simulink model "Assignment_3_simulink"  (R2025a)
settings: Solver=FixedStepDiscrete  StartTime=0.0  StopTime=inf  FixedStep=0.1  RelTol=1e-3  EnableMultiTasking=on
model workspace (MAT data in the model file):
  SL_ROS_VariableLengthArrays_MaxSizes.CommonInfo.ArrayTruncateAction = 'EmitWarning'
  SL_ROS_VariableLengthArrays_MaxSizes.MsgTypeMap = containers.Map
  SL_ROS_VariableLengthArrays_MaxSizes.MsgTypeMap.serialization.keys = {'sensor_msgs/Image', 'sensor_msgs/LaserScan'}
  SL_ROS_VariableLengthArrays_MaxSizes.MsgTypeMap.serialization.values{1}(1).PropertyName = 'data'
  SL_ROS_VariableLengthArrays_MaxSizes.MsgTypeMap.serialization.values{1}(1).DataType = 'uint8'
  SL_ROS_VariableLengthArrays_MaxSizes.MsgTypeMap.serialization.values{1}(1).MaxLength = 921600
  SL_ROS_VariableLengthArrays_MaxSizes.MsgTypeMap.serialization.values{1}(2).PropertyName = 'encoding'
  SL_ROS_VariableLengthArrays_MaxSizes.MsgTypeMap.serialization.values{1}(2).DataType = 'uint8'
  SL_ROS_VariableLengthArrays_MaxSizes.MsgTypeMap.serialization.values{1}(2).MaxLength = 128
  SL_ROS_VariableLengthArrays_MaxSizes.MsgTypeMap.serialization.values{2}(1).PropertyName = 'intensities'
  SL_ROS_VariableLengthArrays_MaxSizes.MsgTypeMap.serialization.values{2}(1).DataType = 'single'
  SL_ROS_VariableLengthArrays_MaxSizes.MsgTypeMap.serialization.values{2}(1).MaxLength = 360
  SL_ROS_VariableLengthArrays_MaxSizes.MsgTypeMap.serialization.values{2}(2).PropertyName = 'ranges'
  SL_ROS_VariableLengthArrays_MaxSizes.MsgTypeMap.serialization.values{2}(2).DataType = 'single'
  SL_ROS_VariableLengthArrays_MaxSizes.MsgTypeMap.serialization.values{2}(2).MaxLength = 360
  SL_ROS_VariableLengthArrays_MaxSizes.MsgTypeMap.serialization.uniformity = 0
  SL_ROS_VariableLengthArrays_MaxSizes.MsgTypeMap.serialization.keyType = 'char'
  SL_ROS_VariableLengthArrays_MaxSizes.MsgTypeMap.serialization.valueType = 'any'
values from neighbouring files (symbols this model uses):
  Kv = 0.8    [Assignment_3.m]
  Kw = 0.3    [Assignment_3.m]
  limit_inf = zeros(1,length(hsv_1))    [Assignment_3.m]
  limit_sup = zeros(1,length(hsv_1))    [Assignment_3.m]
  theta_ref = 1.05*pi    (= 3.29867228627)    [Assignment_3.m]
  toll = 0.001    [Assignment_3.m]
undefined symbols (not defined in the file or in its folder): Rec, SDTV, twist
libraries: ros2lib x6, simulink x3, visionstatistics x1, visionconversions x1, visiontextngfix x1
settings Model: Creator=diego  LastModifiedBy=nicola-bertocchi
settings OptimizationCC: DefaultParameterBehavior=Inlined  EnhancedBackFolding=on  PassReuseOutputArgsAs=Individual arguments  ZeroExternalMemoryAtStartup=off  ZeroInternalMemoryAtStartup=off  MaxStackSize=64  OptimizeBlockOrder=speed  DifferentSizesBufferReuse=on  OptimizationCustomize=off  EfficientTunableParamExpr=on
settings DebuggingCC: ParameterTunabilityLossMsg=error
settings HardwareCC: ProdBitPerLong=64.0  ProdHWDeviceType=Intel->x86-64 (Linux 64)
settings SFSimCC: MATLABDynamicMemAlloc=off
settings RTWCC: SystemTargetFile=ert.tlc  HardwareBoard=Robot Operating System 2 (ROS 2)  TLCOptions="-aInlineSetEventsForThisBaseRateFcn=TLC_FALSE -aSuppressMultiTaskScheduler=TLC_FALSE  -aRateBasedStepFcn=0"  TemplateMakefile=ert_default_tmf  Toolchain=Colcon Tools  TargetLang=C++  Description=Embedded Coder
settings CodeAppCC: ForceParamTrailComments=on  IgnoreCustomStorageClasses=off  OperatorAnnotations=on  SimulinkDataObjDesc=on  SFDataObjDesc=on  InsertBlockDesc=on
settings ERTTargetCC: ExtModeTransport=2.0  ExtModeAutomaticAllocSize=off  RootIOFormat=Structure reference  CodeInterfacePackaging=C++ class

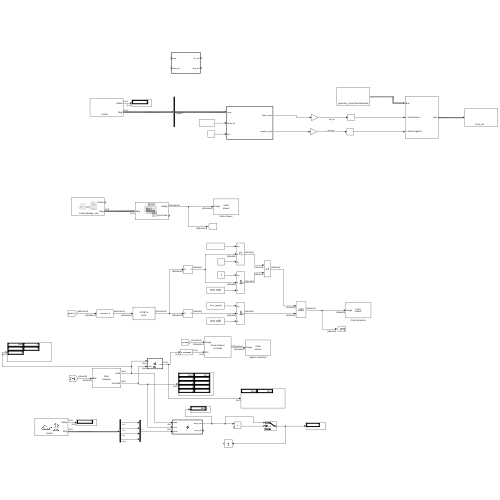
[thumbnail: Simulink's stored preview of the top-level diagram]
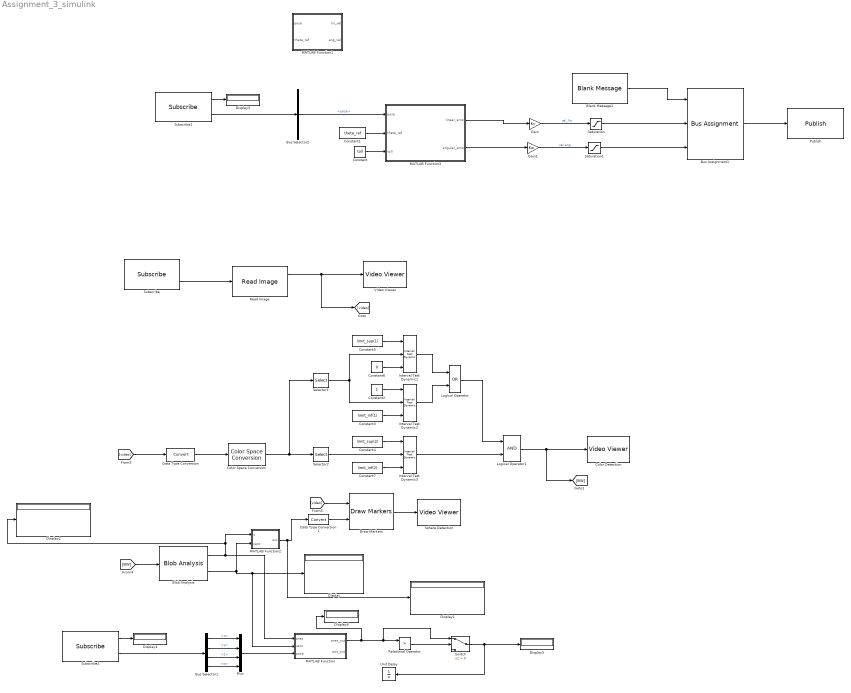
== system Assignment_3_simulink ==
  Blank Message1 : ros2lib/Blank Message  messageClass=Message  entityType=geometry_msgs/TwistStamped  messageType=geometry_msgs/TwistStamped  SampleTime=inf
  Blob Analysis : visionstatistics/Blob Analysis  Tag=vipblks_row_conv  area=on  centroid=on  bBox=off  majorAxis=off  minorAxis=off  angle=off  eccentricity=off  equivDiameterSq=off  extent=off  perimeter=off  outDT=double  conn=8  isLabel=off  maxBlobs=5  warnIfNumBlobsExceeded=on  isCount=off  useMinArea=off  minArea=0  useMaxArea=off  maxArea=intmax('uint32')  excludeBorderBlob=off  isOutVarDim=off  isFill=on  fillValues=-1  roundingMode=Floor  overflowMode=off  prodOutputMode=Binary point scaling  prodOutputWordLength=32  prodOutputFracLength=16  accumMode=Binary point scaling  accumWordLength=32  accumFracLength=0  outputMode=Binary point scaling  outputWordLength=32  outputFracLength=16  firstCoeffMode=Binary point scaling  firstCoeffWordLength=16  firstCoeffFracLength=14  secondCoeffMode=Binary point scaling  secondCoeffWordLength=32  secondCoeffFracLength=16
  Bus Assignment1 : BusAssignment  AssignedSignals=twist.linear.x,twist.angular.z
  Bus Selector1 : BusSelector  OutputSignals=pose.pose.orientation.x,pose.pose.orientation.y,pose.pose.orientation.z,pose.pose.orientation.w
  Bus Selector2 : BusSelector  OutputSignals=pose
  Color Detection : VideoViewer  FigPos=[915 518 418 304]
  Color Space Conversion : visionconversions/Color Space  Conversion  conversion=Obsolete  conversionActive=R'G'B' to HSV  wp_str=D65  rec=Rec. 601 (SDTV)  sys=1125/60/2:1  imagePorts=One multidimensional signal
  Constant : Constant  Value=toll
  Constant1 : Constant  Value=theta_ref
  Constant2 : Constant
  Constant3 : Constant  Value=limit_inf(1)
  Constant4 : Constant  Value=limit_sup(2)
  Constant5 : Constant  Value=limit_sup(1)
  Constant6 : Constant  Value=0
  Constant7 : Constant  Value=limit_inf(2)
  Data Type Conversion : DataTypeConversion  SaturateOnIntegerOverflow=off  RndMeth=Floor
  Data Type Conversion1 : DataTypeConversion  SaturateOnIntegerOverflow=off  RndMeth=Floor
  Display{,1..6} (7 alike) : Display
  Draw Markers : visiontextngfix/Draw Markers  shape=X-mark  size=25  fill=off  fillClrSource=Specify via dialog  display=User-specified value  intensity=200  color=[255 0 0]  opacity=0.6  viewport=Entire image  antialiasing=off  inType=Obsolete  imagePorts=One multidimensional signal  roundingMode=Floor  overflowMode=off  memoryMode=Specify word length  memoryWordLength=16  memoryFracLength=15  prodOutputMode=Binary point scaling  prodOutputWordLength=32  prodOutputFracLength=14
  Gain : Gain  Gain=Kv
  Gain1 : Gain  Gain=Kw
  Interval Test Dynamic1 : simulink/Logic and Bit Operations/Interval Test Dynamic  IntervalClosedRight=on  IntervalClosedLeft=on  OutDataTypeStr=boolean
  Interval Test Dynamic2 : simulink/Logic and Bit Operations/Interval Test Dynamic  IntervalClosedRight=on  IntervalClosedLeft=on  OutDataTypeStr=boolean
  Interval Test Dynamic3 : simulink/Logic and Bit Operations/Interval Test Dynamic  IntervalClosedRight=on  IntervalClosedLeft=on  OutDataTypeStr=boolean
  Logical Operator : Logic  Operator=OR  AllPortsSameDT=off  OutDataTypeStr=boolean
  Logical Operator1 : Logic  AllPortsSameDT=off  OutDataTypeStr=boolean
  MATLAB Function : MATLAB Function  TreatAsAtomicUnit=on
  MATLAB Function1 : MATLAB Function  TreatAsAtomicUnit=on
  MATLAB Function2 : MATLAB Function  TreatAsAtomicUnit=on
  MATLAB Function3 : MATLAB Function  TreatAsAtomicUnit=on
  Mux : Mux
  Publish : ros2lib/Publish  topicSource=Select from ROS network  topic=/cmd_vel  messageType=geometry_msgs/TwistStamped  QOSHistory=Keep last  QOSDepth=10  QOSReliability=Reliable  QOSDurability=Volatile  QOSDeadline=Inf  QOSLifespan=Inf  QOSLiveliness=Automatic  QOSLeaseDuration=Inf  QOSAvoidROSNamespaceConventions=off
  Read Image : ros2lib/Read Image  MaximumImageSize=[480, 640]  ImageEncoding=rgb8  ShowAlphaOutput=off  ShowErrorCodeOutput=on  VariableSizeOutputs=off
  Relational Operator : RelationalOperator  Operator=>  OutDataTypeStr=boolean  RndMeth=Simplest  InputSameDT=off
  Saturation : Saturate  UpperLimit=0.2  LowerLimit=0
  Saturation1 : Saturate  UpperLimit=0.4  LowerLimit=0
  Selector1 : Selector  NumberOfDimensions=3  InputPortWidth=3  IndexOptions=Index vector (dialog),Index vector (dialog),Index vector (dialog)  Indices=[1:480],[1:640],1  OutputSizes=1,1,1
  Selector2 : Selector  NumberOfDimensions=3  InputPortWidth=3  IndexOptions=Index vector (dialog),Index vector (dialog),Index vector (dialog)  Indices=[1:480],[1:640],2  OutputSizes=1,1,1
  Sphere Detection : VideoViewer  FigPos=[795 742 511 303]
  Subscribe : ros2lib/Subscribe  topicSource=Select from ROS network  topic=/camera/image_raw  messageType=sensor_msgs/Image  sampleTime=-1  QOSHistory=Keep last  QOSDepth=10  QOSReliability=Reliable  QOSDurability=Volatile  QOSDeadline=Inf  QOSLifespan=Inf  QOSLiveliness=Automatic  QOSLeaseDuration=Inf  QOSAvoidROSNamespaceConventions=off
  Subscribe1 : ros2lib/Subscribe  topicSource=Select from ROS network  topic=/odom  messageType=nav_msgs/Odometry  sampleTime=-1  QOSHistory=Keep last  QOSDepth=10  QOSReliability=Reliable  QOSDurability=Volatile  QOSDeadline=Inf  QOSLifespan=Inf  QOSLiveliness=Automatic  QOSLeaseDuration=Inf  QOSAvoidROSNamespaceConventions=off
  Subscribe2 : ros2lib/Subscribe  topicSource=Select from ROS network  topic=/odom  messageType=nav_msgs/Odometry  sampleTime=-1  QOSHistory=Keep last  QOSDepth=10  QOSReliability=Reliable  QOSDurability=Volatile  QOSDeadline=Inf  QOSLifespan=Inf  QOSLiveliness=Automatic  QOSLeaseDuration=Inf  QOSAvoidROSNamespaceConventions=off
  Switch : Switch  Criteria=u2 > Threshold  SaturateOnIntegerOverflow=off  InputSameDT=off
  Unit Delay : UnitDelay  SampleTime=-1  HasFrameUpgradeWarning=on
  Video Viewer : VideoViewer  FigPos=[155 894 418 304]
  wires:
  Subscribe/2 -> Read Image/1
  Read Image/1 -> Video Viewer/1, [video]
  [video] -> Data Type Conversion/1
  Data Type Conversion/1 -> Color Space Conversion/1
  Color Space Conversion/1 -> Selector1/1, Selector2/1
  [BW] -> Blob Analysis/1
  Blob Analysis/1 -> MATLAB Function2/1(u), Display2/1, MATLAB Function/1(area)
  MATLAB Function2/1(out) -> Display1/1, Data Type Conversion1/1
  Blob Analysis/2 -> MATLAB Function/2(cent), Display/1, MATLAB Function2/2(cent)
  Data Type Conversion1/1 -> Draw Markers/2
  [video] -> Draw Markers/1
  Draw Markers/1 -> Sphere Detection/1
  Bus Assignment1/1 -> Publish/1
  Gain/1 -> Saturation/1  "vel_lin"
  Gain1/1 -> Saturation1/1  "vel ang"
  Saturation1/1 -> Bus Assignment1/3
  Subscribe1/1 -> Display3/1
  Saturation/1 -> Bus Assignment1/2
  Subscribe1/2 -> Bus Selector2/1
  Bus Selector2/1 -> MATLAB Function3/1(pose)  "<pose>"
  Blank Message1/1 -> Bus Assignment1/1
  Constant1/1 -> MATLAB Function3/2(theta_ref)
  MATLAB Function3/1(linear_error) -> Gain/1
  MATLAB Function3/2(angular_error) -> Gain1/1
  Constant6/1 -> Interval Test Dynamic1/3
  Constant5/1 -> Interval Test Dynamic1/1
  Constant2/1 -> Interval Test Dynamic2/1
  Constant3/1 -> Interval Test Dynamic2/3
  Interval Test Dynamic1/1 -> Logical Operator/1
  Interval Test Dynamic2/1 -> Logical Operator/2
  Selector1/1 -> Interval Test Dynamic1/2, Interval Test Dynamic2/2
  Constant7/1 -> Interval Test Dynamic3/3
  Constant4/1 -> Interval Test Dynamic3/1
  Selector2/1 -> Interval Test Dynamic3/2
  Logical Operator/1 -> Logical Operator1/1
  Logical Operator1/1 -> [BW], Color Detection/1
  Interval Test Dynamic3/1 -> Logical Operator1/2
  Constant/1 -> MATLAB Function3/3(toll)
  Subscribe2/1 -> Display4/1
  Subscribe2/2 -> Bus Selector1/1
  MATLAB Function/1(area_out) -> Display6/1, Switch/1, Relational Operator/1
  Relational Operator/1 -> Switch/2
  Switch/1 -> Display5/1, Unit Delay/1
  Bus Selector1/1 -> Mux/1  "<x>"
  Bus Selector1/2 -> Mux/2  "<y>"
  Bus Selector1/3 -> Mux/3  "<z>"
  Bus Selector1/4 -> Mux/4  "<w>"
  Mux/1 -> MATLAB Function/3(pose)

== matlab function Assignment_3_simulink/MATLAB Function2 ==
  data: u input; out output; cent input
function out = fcn(u,cent)

[~,i] = max(u);

if ~isempty(i)
    out=cent(i,:);
else
    out=[0,0];

end

== matlab function Assignment_3_simulink/MATLAB Function ==
  data: area input; cent input; area_out output; pose input; pos_out output
function [area_out,pos_out] = fcn(area,cent,pose)

area_out = 0;
pos_out = zeros(size(pose));
[val,i] = max(area);    

if val~=-1
    if ~isempty(i)
        if cent(i,1)>315 && cent(i,1)<325
            area_out = double(val);
            pos_out = pose;
        end
    end 
end

== matlab function Assignment_3_simulink/MATLAB Function3 ==
  data: linear_error output; pose input; theta_ref input; toll input; angular_error output
function [linear_error, angular_error] = Interruttore(pose, theta_ref, toll)
    
  
 %   angular_error = 0; % Valore di default (risolve l'errore Coder)
linear_error = 0;
    q_current = [pose.pose.orientation.x; 
                 pose.pose.orientation.y; 
                 pose.pose.orientation.z; 
                 pose.pose.orientation.w];
             
% 1. Definisci l'input (Yaw, Pitch, Roll)
eul = [theta_ref, 0, 0]; 

% 2. Chiama la funzione. L'output è [w, x, y, z]
q_matlab = eul2quat(eul); 

% 3. Riordina l'output nel formato ROS [x, y, z, w]
q_target = [q_matlab(2);   % x
            q_matlab(3);   % y
            q_matlab(4);   % z
            q_matlab(1)];  % w

           
       % ... (Calcolo del quaternione di errore, come prima) ...
       q_current_inv = [-q_current(1); -q_current(2); -q_current(3); q_current(4)];
       x1 = q_target(1); y1 = q_target(2); z1 = q_target(3); w1 = q_target(4);
       x2 = q_current_inv(1); y2 = q_current_inv(2); z2 = q_current_inv(3); w2 = q_current_inv(4);
       q_error = zeros(4, 1);
       q_error(4) = w1*w2 - x1*x2 - y1*y2 - z1*z2; % W
       q_error(1) = w1*x2 + x1*w2 + y1*z2 - z1*y2; % X
       q_error(2) = w1*y2 - x1*z2 + y1*w2 + z1*x2; % Y
       q_error(3) = w1*z2 + x1*y2 - y1*x2 + z1*w2; % Z
       
       angular_error = norm(q_error(1:3)); 
       
      
       % if angular_error < deg2rad(toll)
       %       angular_error = 0; 
       % end
end

== matlab function Assignment_3_simulink/MATLAB Function1 ==
  data: pose input; lin_vel output; theta_ref input; ang_vel output
function [lin_vel,ang_vel] = control(pose,theta_ref)
  % 1. Ignoriamo "pose":
  % Dato che vuoi ruotare all'infinito, non ci interessa l'orientamento 
  % attuale del robot (q_current). Lui deve girare a prescindere.

  % 2. Impostiamo le velocità dirette:
  lin_vel = 0;          % Fermo sul posto (nessun movimento in avanti)
  ang_vel = 0.4;  % La velocità di rotazione è ESATTAMENTE il valore in ingresso
end
